simulink model "close_loop_tf2"  (R2017a)
settings: Solver=VariableStepAuto  StartTime=0.0  StopTime=T  RelTol=1e-3
values from neighbouring files (symbols this model uses):
  seed = randi([0 1000],1)    [close_loop_step_dg.m]    (also in close_loop_tf2_dg.m; multi_sin_damp_dg.m; open_loop_step_dg.m; open_noise_dg.m)
  tau = 50    [testbench.m]
  Ts = 1/Fs    (= 0.01)    [close_loop_step_dg.m]    (also in close_loop_tf2_dg.m = 0.001; open_loop_step_dg.m; testbench.m)
libraries: simulink x2
settings Model: Creator=ljxia_000  LastModifiedBy=ljxia

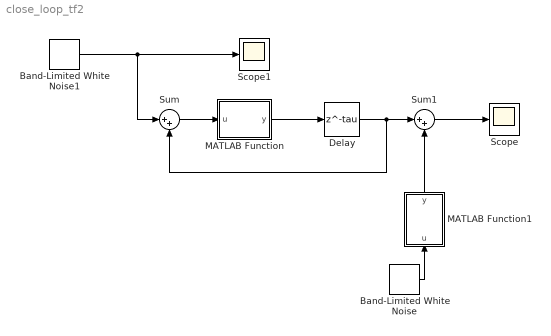
== system close_loop_tf2 ==
  Band-Limited White Noise : simulink/Sources/Band-Limited White Noise  Cov=[0.1]  Ts=Ts  seed=[seed]
  Band-Limited White Noise1 : simulink/Sources/Band-Limited White Noise  Cov=[0.1]  Ts=Ts  seed=[seed+1]
  Delay : Delay  DelayLength=tau  InitialCondition=0  SampleTime=Ts
  MATLAB Function : MATLAB Function  TreatAsAtomicUnit=on
  MATLAB Function1 : MATLAB Function  TreatAsAtomicUnit=on
  Scope : Scope
  Scope1 : Scope
  Sum : Sum  Inputs=|++
  Sum1 : Sum  Inputs=|++
  wires:
  Sum/1 -> MATLAB Function/1(u)
  MATLAB Function/1(y) -> Delay/1
  Delay/1 -> Sum/2, Sum1/1
  Sum1/1 -> Scope/1
  Band-Limited White Noise/1 -> MATLAB Function1/1(u)
  MATLAB Function1/1(y) -> Sum1/2
  Band-Limited White Noise1/1 -> Sum/1, Scope1/1

== matlab function close_loop_tf2/MATLAB Function1 ==
  data: u input; y output
function y = fcn(u)
y = 0.71/(1-0.7*u^-1);

== matlab function close_loop_tf2/MATLAB Function ==
  data: u input; y output
function y = fcn(u)
Ts = 100;
y = 0.6*(1+Ts/50 -u^-1)/(1-u^-1);
